simulink model "gettingstartedwithethercat"  (R2016b)
settings: Solver=FixedStepDiscrete  StartTime=0.0  StopTime=inf  FixedStep=0.01  RelTol=1e-3  EnableMultiTasking=on
libraries: xpcethercatlib x5, slrtlib x3
settings Model: xpc_rtwmakecfg_data=_xpcethercatlib_  SimulationMode=external  Creator=march  LastModifiedBy=march
settings SolverCC: EnableConcurrentExecution=on
settings DataIOCC: SaveFormat=StructureWithTime
settings OptimizationCC: BlockReduction=off  OptimizeBlockIOStorage=off  BufferReuse=off  GlobalBufferReuse=off  ExpressionFolding=off  LocalBlockOutputs=off
settings HardwareCC: ProdBitPerPointer=32  ProdBitPerSizeT=32  ProdBitPerPtrDiffT=32  ProdLargestAtomicFloat=None  ProdWordSize=32  ProdLongLongMode=on  ProdHWDeviceType=Generic->32-bit x86 compatible
settings RTWCC: SystemTargetFile=slrt.tlc  TemplateMakefile=slrt_default_tmf  Description=Simulink Real-Time  RTWCompilerOptimization=on

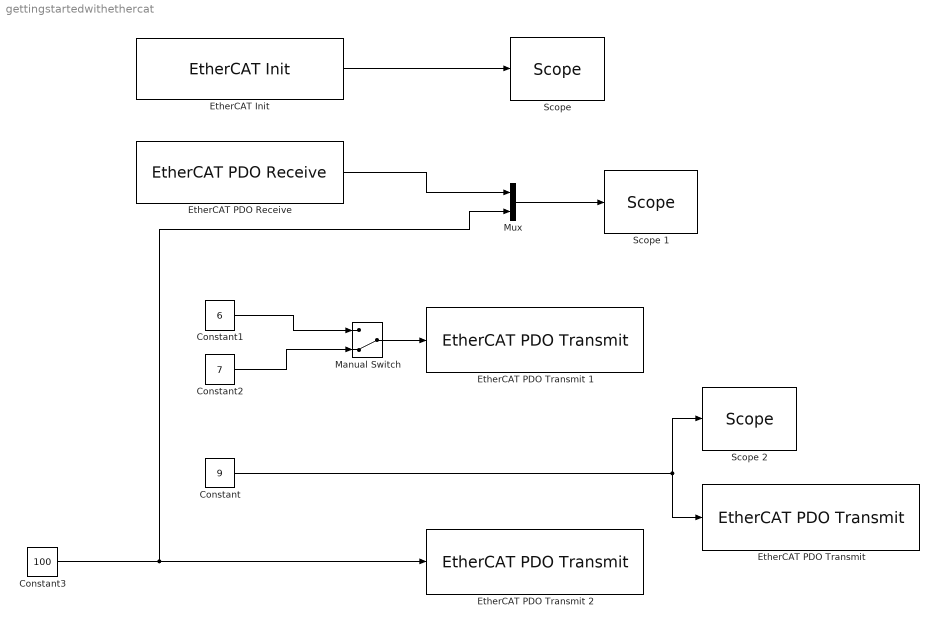
== system gettingstartedwithethercat ==
  Constant : Constant  Value=9  OutDataTypeStr=int8
  Constant1 : Constant  Value=6  OutDataTypeStr=uint16
  Constant2 : Constant  Value=7  OutDataTypeStr=uint16
  Constant3 : Constant  Value=100  OutDataTypeStr=int32
  "EtherCAT Init " : xpcethercatlib/EtherCAT Init   Priority=0  config_file=D:\CloudStation\2016-2017\03-Tech\04-Software & Control\Simulink Models\somanet.xml  device_id=0  pci_bus=3  pci_slot=0  dctuning=1  enaDebug=off  enaDC=on  errLink=off  masterDbg=off  stateChgDbg=off  baseClock=off  masterCfg=off  logFile='c:\dbglog.txt'  sample_time=0.010000  DCMode=0
  EtherCAT PDO Receive : xpcethercatlib/EtherCAT PDO Receive  Priority=2  sig_name=Box 1 (Synapticon-ECAT).Tx PDO Mapping.Velocity Value  sig_offset=264  sig_type=int32  type_size=32  sig_dim=1  device_id=0  sample_time=0.010000
  "EtherCAT PDO Transmit " : xpcethercatlib/EtherCAT PDO Transmit   Priority=3  sig_name=Box 1 (Synapticon-ECAT).Rx PDO Mapping.Op Mode  sig_offset=224  sig_type=int8  type_size=8  sig_dim=1  device_id=0  sample_time=0.010000
  EtherCAT PDO Transmit 1 : xpcethercatlib/EtherCAT PDO Transmit   Priority=3  sig_name=Box 1 (Synapticon-ECAT).Rx PDO Mapping.Controlword  sig_offset=208  sig_type=uint16  type_size=16  sig_dim=1  device_id=0  sample_time=0.010000
  EtherCAT PDO Transmit 2 : xpcethercatlib/EtherCAT PDO Transmit   Priority=3  sig_name=Box 1 (Synapticon-ECAT).Rx PDO Mapping.Target Velocity  sig_offset=280  sig_type=int32  type_size=32  sig_dim=1  device_id=0  sample_time=0.010000
  Manual Switch : ManualSwitch  CurrentSetting=0
  Mux : Mux  Inputs=2
  "Scope " : slrtlib/Displays and Logging/Scope   scopeno=1  scopetype=Target  autostart=on  viewmode=Graphical redraw  formatstr='%15.6f'  grid=on  ylimits=[0,0]  nosamples=250  noprepostsamples=0  interleave=1  triggermode=FreeRun  triggersignal=1  trigsignalfromport=off  triggerlevel=0.0  triggerslope=Either  triggerscope=1  triggersample=0  filename=data.dat  mode=Lazy  writesize=512  autorestart=off  dynamicfilemode=off  maxwritefilesize=512*1024^2
  Scope 1 : slrtlib/Displays and Logging/Scope   scopeno=2  scopetype=Target  autostart=on  viewmode=Graphical sliding  formatstr='%15.6f'  grid=on  ylimits=[0,200]  nosamples=250  noprepostsamples=0  interleave=1  triggermode=FreeRun  triggersignal=1  trigsignalfromport=off  triggerlevel=0.0  triggerslope=Either  triggerscope=1  triggersample=0  filename=data.dat  mode=Lazy  writesize=512  autorestart=off  dynamicfilemode=off  maxwritefilesize=512*1024^2
  Scope 2 : slrtlib/Displays and Logging/Scope   scopeno=3  scopetype=Target  autostart=on  viewmode=Graphical redraw  formatstr='%15.6f'  grid=on  ylimits=[0,0]  nosamples=250  noprepostsamples=0  interleave=1  triggermode=FreeRun  triggersignal=1  trigsignalfromport=off  triggerlevel=0.0  triggerslope=Either  triggerscope=1  triggersample=0  filename=data.dat  mode=Lazy  writesize=512  autorestart=off  dynamicfilemode=off  maxwritefilesize=512*1024^2
  wires:
  "EtherCAT Init "/1 -> "Scope "/1
  Manual Switch/1 -> EtherCAT PDO Transmit 1/1
  Constant1/1 -> Manual Switch/1
  Constant2/1 -> Manual Switch/2
  Constant/1 -> "EtherCAT PDO Transmit "/1, Scope 2/1
  Constant3/1 -> EtherCAT PDO Transmit 2/1, Mux/2
  EtherCAT PDO Receive/1 -> Mux/1
  Mux/1 -> Scope 1/1
